simulink model "Models_for_report"  (R2015b)
settings: Solver=VariableStepAuto  StartTime=0.0  StopTime=10.0  RelTol=1e-3
undefined symbols (not defined in the file): C_drag, J_pro, Kt, Kv, R, T_L, TS, Vin
settings Model: Creator=Morten  LastModifiedBy=Morten

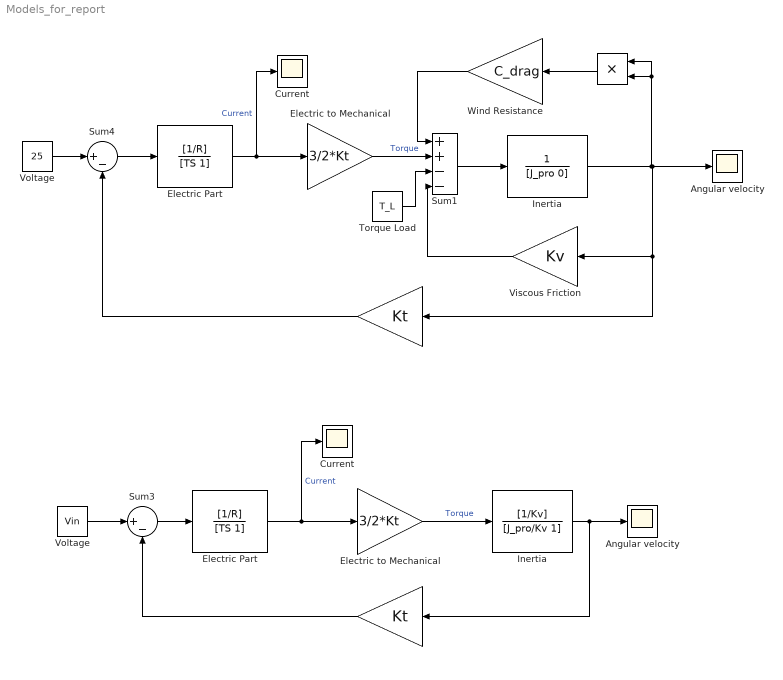
== system Models_for_report ==
  "           " : Product
  "            " : Gain  Gain=Kt
  "             " : Gain  Gain=Kt
  Angular velocity : Scope
  "Angular velocity " : Scope
  Current : Scope
  "Current " : Scope
  Electric Part : TransferFcn  Numerator=[1/R]  Denominator=[TS 1]
  "Electric Part " : TransferFcn  Numerator=[1/R]  Denominator=[TS 1]
  Electric to Mechanical : Gain  Gain=3/2*Kt
  "Electric to Mechanical " : Gain  Gain=3/2*Kt
  Inertia : TransferFcn  Denominator=[J_pro 0]
  "Inertia " : TransferFcn  Numerator=[1/Kv]  Denominator=[J_pro/Kv 1]
  Sum1 : Sum  Inputs=++--
  Sum3 : Sum  Inputs=|+-
  Sum4 : Sum  Inputs=|+-
  Torque Load : Constant  Value=T_L
  Viscous Friction : Gain  Gain=Kv
  Voltage : Constant  Value=25
  "Voltage " : Constant  Value=Vin
  Wind Resistance : Gain  Gain=C_drag
  wires:
  "            "/1 -> Sum4/2
  Sum4/1 -> Electric Part/1
  Electric Part/1 -> Current/1, Electric to Mechanical/1  "Current"
  "           "/1 -> Wind Resistance/1
  Voltage/1 -> Sum4/1
  Electric to Mechanical/1 -> Sum1/2  "Torque"
  Sum1/1 -> Inertia/1
  Wind Resistance/1 -> Sum1/1
  Torque Load/1 -> Sum1/3
  Viscous Friction/1 -> Sum1/4
  Inertia/1 -> Angular velocity/1, Viscous Friction/1, "            "/1, "           "/1, "           "/2
  "             "/1 -> Sum3/2
  Sum3/1 -> "Electric Part "/1
  "Electric Part "/1 -> "Current "/1, "Electric to Mechanical "/1  "Current"
  "Voltage "/1 -> Sum3/1
  "Electric to Mechanical "/1 -> "Inertia "/1  "Torque"
  "Inertia "/1 -> "Angular velocity "/1, "             "/1
